simulink library "CryoDetLibCMB"  (R2016b)
settings: Solver=VariableStepAuto  StartTime=0.0  StopTime=10.0  RelTol=1e-3
values from neighbouring files (symbols this model uses):
  Fclk = Fadc    (= 307200000)    [setupCryoFPGA.m]    (also in setupCryoFPGA_CMB.m; setupCryoFPGAorig.m = 312500000)
undefined symbols (not defined in the file or in its folder): xlipgetpartsetting
libraries: xbsIndex_r4 x255, CryoDetLibCMB x19, CryoDetLib x2, simulink x1
(part 2 of 3)

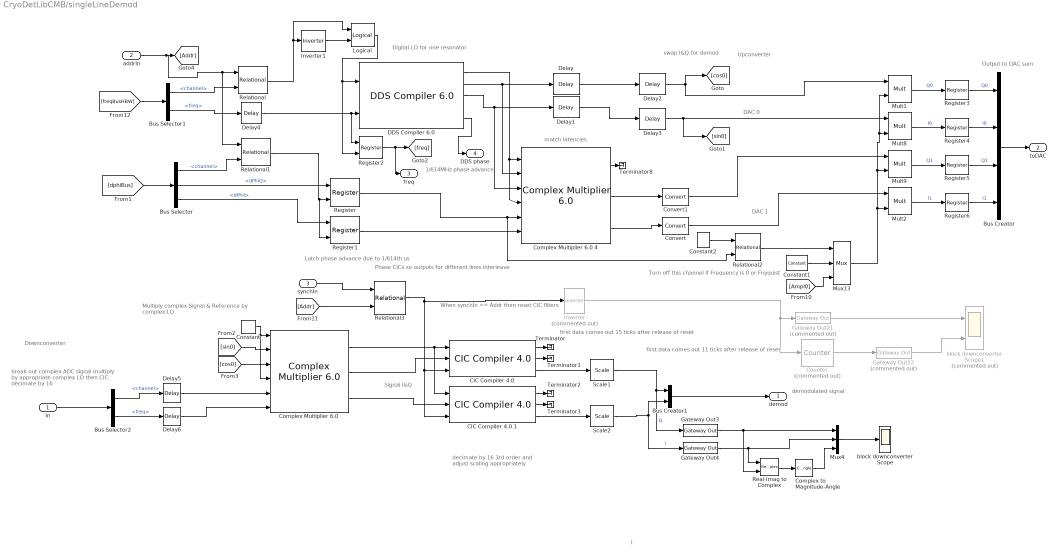
== system CryoDetLibCMB/singleLineDemod ==
  note: swap I&Q for demod
  note: Output to DAC sum
  note: decimate by 16 3rd order
      | and adjust scaling appropriately
  note: When synchIn == Addr then reset CIC filters
  note: Turn off this channel if Frequency is 0 or Fnyquist
  note: first data comes out 15 ticks after release of reset
  note: Latch phase advance due to 1/614th us
  note: I
  note: DAC 1
  note: DAC 0
  note: Downconverter
  note: demodulated signal
  note: Phase CICs so outputs for different lines interleave
  note: Signal I&Q
  note: Multiply complex Signal & Reference
      | by complex LO
  note: match latencies
  note: 1/614MHz
      | phase advance
  note: break out complex ADC signal
      | multiply by appropriate complex LO
      | then CIC decimate by 16
  note: Digital LO for one resonator
  note: Upconverter
  note: first data comes out 11 ticks after release of reset
  In : Inport
  addrIn : Inport  Port=2
  synchIn : Inport  Port=3
  Bus Creator : BusCreator  Inputs=4
  Bus Creator1 : BusCreator  Inputs=2
  Bus Selector : BusSelector  OutputSignals=channel,dPhiQ,dPhiI
  Bus Selector1 : BusSelector  OutputSignals=channel,freq
  Bus Selector2 : BusSelector  OutputSignals=channel,freq
  "CIC Compiler 4.0 " : xbsIndex_r4/CIC Compiler 4.0   filter_type=Decimation  number_of_stages=3  differential_delay=1  number_of_channels=1  sample_rate_changes=Fixed  fixed_or_initial_rate=16  minimum_rate=16  maximum_rate=16  ratespecification=Sample_Period  sampleperiod=1  hardwareoversamplingrate=1  quantization=Truncation  output_data_width=20  use_xtreme_dsp_slice=off  use_streaming_interface=on  has_aclken=off  has_aresetn=on  has_dout_tready=off  trim_axipin_name=on  gui_behaviour=Sysgen_GUI  input_data_width=18  ip_name=CIC Compiler  ip_version=4.0  dsptool_ready=true  wrapper_available=true  port_translation_map={ 'aclken' => 'en', 'aresetn' => 'rst' }  ipcore_xco_need_fpga_part=true  ipcore_verbose=false  block_type=cic_compiler_v4_0
  CIC Compiler 4.0 1 : xbsIndex_r4/CIC Compiler 4.0   filter_type=Decimation  number_of_stages=3  differential_delay=1  number_of_channels=1  sample_rate_changes=Fixed  fixed_or_initial_rate=16  minimum_rate=16  maximum_rate=16  ratespecification=Sample_Period  sampleperiod=1  hardwareoversamplingrate=1  quantization=Truncation  output_data_width=20  use_xtreme_dsp_slice=off  use_streaming_interface=on  has_aclken=off  has_aresetn=on  has_dout_tready=off  trim_axipin_name=on  gui_behaviour=Sysgen_GUI  input_data_width=18  ip_name=CIC Compiler  ip_version=4.0  dsptool_ready=true  wrapper_available=true  port_translation_map={ 'aclken' => 'en', 'aresetn' => 'rst' }  ipcore_xco_need_fpga_part=true  ipcore_verbose=false  block_type=cic_compiler_v4_0
  "Complex Multiplier 6.0 " : xbsIndex_r4/Complex Multiplier 6.0   hasatlast=off  hasatuser=off  atuserwidth=1  hasbtlast=off  hasbtuser=off  btuserwidth=1  multtype=Use_Mults  optimizegoal=Resources  flowcontrol=NonBlocking  outputwidth=18  roundmode=Truncate  hasctrltlast=off  hasctrltuser=off  ctrltuserwidth=1  outtlastbehv=Null  latencyconfig=Automatic  minimumlatency=37  aclken=off  aresetn=off  trim_axipin_name=on  simulation_type=hybrid_sim  simulation_model=sysgen:cmpy_v6_0  data_path_portlist={ 's_axis_a_tdata_real', 's_axis_a_tdata_imag', 's_axis_b_tdata_real', 's_axis_b_tdata_imag', 's_axis_ctrl_tdata_rounding_bit', 'm_axis_dout_tdata_real', 'm_axis_dout_tdata_imag' }  aportwidth=63  bportwidth=63  ip_name=Complex Multiplier  ip_version=6.0  dsptool_ready=true  ipcore_usecache=true  ipcore_useipmodelcache=true  ipcore_verbose=false  ipcore_latency_parameter='minimumlatency'  wrapper_available=true  port_translation_map={ 'aclken' => 'en', 'aresetn' => 'rst'}  block_type=cmpy_v6_0
  Complex Multiplier 6.0 4 : xbsIndex_r4/Complex Multiplier 6.0   hasatlast=off  hasatuser=off  atuserwidth=1  hasbtlast=off  hasbtuser=off  btuserwidth=1  multtype=Use_Mults  optimizegoal=Resources  flowcontrol=NonBlocking  outputwidth=19  roundmode=Truncate  hasctrltlast=off  hasctrltuser=off  ctrltuserwidth=1  outtlastbehv=Null  latencyconfig=Manual  minimumlatency=6  aclken=off  aresetn=off  trim_axipin_name=on  simulation_type=hybrid_sim  simulation_model=sysgen:cmpy_v6_0  data_path_portlist={ 's_axis_a_tdata_real', 's_axis_a_tdata_imag', 's_axis_b_tdata_real', 's_axis_b_tdata_imag', 's_axis_ctrl_tdata_rounding_bit', 'm_axis_dout_tdata_real', 'm_axis_dout_tdata_imag' }  aportwidth=63  bportwidth=63  ip_name=Complex Multiplier  ip_version=6.0  dsptool_ready=true  ipcore_usecache=true  ipcore_useipmodelcache=true  ipcore_verbose=false  ipcore_latency_parameter='minimumlatency'  wrapper_available=true  port_translation_map={ 'aclken' => 'en', 'aresetn' => 'rst'}  block_type=cmpy_v6_0
  Complex to Magnitude-Angle : ComplexToMagnitudeAngle  Output=Magnitude
  Constant : xbsIndex_r4/Constant  const=1  gui_display_data_type=Boolean  arith_type=Boolean  n_bits=16  bin_pt=14  preci_type=Single  exp_width=8  frac_width=24  explicit_period=off  period=1  equ=P=C  opselect=C  inp2=PCIN>>17  opr=+  inp1=P  carry=CIN  dbl_ovrd=off  block_type=constant
  Constant1 : xbsIndex_r4/Constant  const=0  gui_display_data_type=Fixed-point  arith_type=Unsigned  n_bits=16  bin_pt=16  preci_type=Single  exp_width=8  frac_width=24  explicit_period=off  period=1  equ=P=C  opselect=C  inp2=PCIN>>17  opr=+  inp1=P  carry=CIN  dbl_ovrd=off  block_type=constant
  Constant2 : xbsIndex_r4/Constant  const=0  gui_display_data_type=Fixed-point  arith_type=Unsigned  n_bits=16  bin_pt=16  preci_type=Single  exp_width=8  frac_width=24  explicit_period=off  period=1  equ=P=C  opselect=C  inp2=PCIN>>17  opr=+  inp1=P  carry=CIN  dbl_ovrd=off  block_type=constant
  Convert : xbsIndex_r4/Convert  gui_display_data_type=Fixed-point  arith_type="Signed  (2's comp)"  n_bits=16  bin_pt=14  float_type=Single  exp_bits=8  fraction_bits=24  quantization=Truncate  overflow=Saturate  en=off  latency=1  pipeline=off  dbl_ovrd=off  block_type=convert
  Convert1 : xbsIndex_r4/Convert  gui_display_data_type=Fixed-point  arith_type="Signed  (2's comp)"  n_bits=16  bin_pt=14  float_type=Single  exp_bits=8  fraction_bits=24  quantization=Truncate  overflow=Saturate  en=off  latency=1  pipeline=off  dbl_ovrd=off  block_type=convert
  Counter : xbsIndex_r4/Counter  Commented=on  cnt_type=Free Running  cnt_to=Inf  operation=Up  start_count=0  cnt_by_val=2^-8  arith_type=Unsigned  n_bits=8  bin_pt=8  load_pin=off  rst=on  en=off  explicit_period=off  period=1  use_behavioral_HDL=off  implementation=Fabric  dbl_ovrd=off  block_type=counter
  "DDS Compiler 6.0 " : xbsIndex_r4/DDS Compiler 6.0   partspresent=Phase_Generator_and_SIN_COS_LUT  dds_clock_rate=Fclk/1e6  channels=1  mode_of_operation=Standard  modulus=9  parameter_entry=Hardware_Parameters  spurious_free_dynamic_range=45  frequency_resolution=0.4  noise_shaping=None  phase_width=freqBits  output_width=IQbits  output_selection=Sine_and_Cosine  negative_sine=off  negative_cosine=off  amplitude_mode=Unit_Circle  memory_type=Auto  optimization_goal=Speed  dsp48_use=Maximal  resync=off  latency_configuration=Configurable  latency=15  has_phase_out=on  has_aclken=off  has_aresetn=off  explicit_period=on  period=Tclk  data_has_tlast=Not_Required  has_tready=off  s_phase_has_tuser=Not_Required  m_data_has_tuser=Not_Required  m_phase_has_tuser=Not_Required  s_phase_tuser_width=1  output_form=Twos_Complement  s_config_sync_mode=On_Vector  phase_increment=Programmable  output_frequency1=0  output_frequency2=0  output_frequency3=0  output_frequency4=0  output_frequency5=0  output_frequency6=0  output_frequency7=0  output_frequency8=0  output_frequency9=0  output_frequency10=0  output_frequency11=0  output_frequency12=0  output_frequency13=0  output_frequency14=0  output_frequency15=0  output_frequency16=0  pinc1='0'  pinc2='0'  pinc3='0'  pinc4='0'  pinc5='0'  pinc6='0'  pinc7='0'  pinc8='0'  pinc9='0'  pinc10='0'  pinc11='0'  pinc12='0'  pinc13='0'  pinc14='0'  pinc15='0'  pinc16='0'  phase_offset=None  phase_offset_angles1=0  phase_offset_angles2=0  phase_offset_angles3=0  phase_offset_angles4=0  phase_offset_angles5=0  phase_offset_angles6=0  phase_offset_angles7=0  phase_offset_angles8=0  phase_offset_angles9=0  phase_offset_angles10=0  phase_offset_angles11=0  phase_offset_angles12=0  phase_offset_angles13=0  phase_offset_angles14=0  phase_offset_angles15=0  phase_offset_angles16=0  poff1='0'  poff2='0'  poff3='0'  poff4='0'  poff5='0'  poff6='0'  poff7='0'  poff8='0'  poff9='0'  poff10='0'  poff11='0'  poff12='0'  poff13='0'  poff14='0'  poff15='0'  poff16='0'  trim_axipin_name=on  simulation_type=hybrid_sim  simulation_model=sysgen:xddsv6_0_cmodel  data_path_portlist={ 's_axis_config_tdata_poff', 's_axis_config_tdata_chan0_poff', 's_axis_config_tdata_pinc', 's_axis_config_tdata_chan0_pinc', 's_axis_phase_tdata_resync', 's_axis_phase_tdata_chan0_resync', 's_axis_phase_tdata_poff', 's_axis_phase_tdata_chan0_poff', 's_axis_phase_tdata_pinc', 's_axis_phase_tdata_chan0_pinc', 's_axis_phase_tdata_phase_in', 'm_axis_data_tdata_sine', 'm_axis_data_tdata_chan0_sine', 'm_axis_data_tdata_cosine', 'm_axis_data_tdata_chan0_cosine', 'm_axis_phase_tdata_phase_out', 'm_axis_phase_tdata_chan0_phase_out'}  por_mode=false  gui_behaviour=Sysgen  ip_name=DDS Compiler  ip_version=6.0  dsptool_ready=true  wrapper_available=true  port_translation_map={ 'aclken' => 'en', 'aresetn' => 'rst' }  ipcore_usecache=true  ipcore_useipmodelcache=true  ipcore_xco_need_fpga_part=true  ipcore_fpga_part=xlipgetpartsetting(gcb, {'kintex7', 'xc7k325t', '-3', 'fbg676'})  ipcore_verbose=false  block_type=dds_compiler_v6_0
  Delay : xbsIndex_r4/Delay  rst=off  infoeditControl=Selection of Reset will increase slice count due to use of real FFs and instead of SRLs  en=off  latency=6  reg_retiming=off  dbl_ovrd=off  block_type=delay
  Delay1 : xbsIndex_r4/Delay  rst=off  infoeditControl=Selection of Reset will increase slice count due to use of real FFs and instead of SRLs  en=off  latency=6  reg_retiming=off  dbl_ovrd=off  block_type=delay
  Delay2 : xbsIndex_r4/Delay  rst=off  infoeditControl=Selection of Reset will increase slice count due to use of real FFs and instead of SRLs  en=off  latency=1  reg_retiming=off  dbl_ovrd=off  block_type=delay
  Delay3 : xbsIndex_r4/Delay  rst=off  infoeditControl=Selection of Reset will increase slice count due to use of real FFs and instead of SRLs  en=off  latency=1  reg_retiming=off  dbl_ovrd=off  block_type=delay
  Delay4 : xbsIndex_r4/Delay  rst=off  infoeditControl=Selection of Reset will increase slice count due to use of real FFs and instead of SRLs  en=off  latency=2  reg_retiming=on  dbl_ovrd=off  block_type=delay
  Delay5 : xbsIndex_r4/Delay  rst=off  infoeditControl=Selection of Reset will increase slice count due to use of real FFs and instead of SRLs  en=off  latency=2  reg_retiming=on  dbl_ovrd=off  block_type=delay
  Delay6 : xbsIndex_r4/Delay  rst=off  infoeditControl=Selection of Reset will increase slice count due to use of real FFs and instead of SRLs  en=off  latency=2  reg_retiming=on  dbl_ovrd=off  block_type=delay
  Gateway Out21 : xbsIndex_r4/Gateway Out  Commented=on  inherit_from_input=off  hdl_port=off  rows=1  columns=1  UseAsDAC=off  DACChannel='1'  interface=None  automatic_assignment=on  address_offset=hex2dec('00')  intf_name=''  intf_description=''  timing_constraint=None  locs_specified=off  LOCs={}  io_standard={}  block_type=gatewayout
  Gateway Out22 : xbsIndex_r4/Gateway Out  Commented=on  inherit_from_input=off  hdl_port=off  rows=1  columns=1  UseAsDAC=off  DACChannel='1'  interface=None  automatic_assignment=on  address_offset=hex2dec('00')  intf_name=''  intf_description=''  timing_constraint=None  locs_specified=off  LOCs={}  io_standard={}  block_type=gatewayout
  Gateway Out3 : xbsIndex_r4/Gateway Out  inherit_from_input=off  hdl_port=off  rows=1  columns=1  UseAsDAC=off  DACChannel='1'  interface=None  automatic_assignment=on  address_offset=hex2dec('00')  intf_name=''  intf_description=''  timing_constraint=None  locs_specified=off  LOCs={}  io_standard={}  block_type=gatewayout
  Gateway Out4 : xbsIndex_r4/Gateway Out  inherit_from_input=off  hdl_port=off  rows=1  columns=1  UseAsDAC=off  DACChannel='1'  interface=None  automatic_assignment=on  address_offset=hex2dec('00')  intf_name=''  intf_description=''  timing_constraint=None  locs_specified=off  LOCs={}  io_standard={}  block_type=gatewayout
  Inverter : xbsIndex_r4/Inverter  Commented=on  en=off  latency=0  dbl_ovrd=off  block_type=inv
  Inverter1 : xbsIndex_r4/Inverter  en=off  latency=1  dbl_ovrd=off  block_type=inv
  Logical : xbsIndex_r4/Logical  logical_function=AND  inputs=2  en=off  latency=1  precision=Full  arith_type=Unsigned  n_bits=16  bin_pt=0  align_bp=on  dbl_ovrd=off  block_type=logical
  Mult{1..2,8..9} (4 alike) : xbsIndex_r4/Mult  precision=User Defined  arith_type="Signed  (2's comp)"  n_bits=16  bin_pt=15  quantization=Truncate  overflow=Wrap  en=off  latency=3  use_behavioral_HDL=off  opt=Speed  use_embedded=on  optimum_pipeline=off  pipeline=on  dbl_ovrd=off  use_rpm=on  placement_style=Triangular  block_type=mult
  Mux13 : xbsIndex_r4/Mux  inputs=2  en=off  latency=0  precision=Full  arith_type=Unsigned  n_bits=16  bin_pt=14  quantization=Truncate  overflow=Wrap  dbl_ovrd=off  block_type=mux
  Mux4 : Mux  Inputs=3
  Real-Imag to Complex : RealImagToComplex
  Register : xbsIndex_r4/Register  init=0  rst=off  en=on  dbl_ovrd=off  block_type=register
  Register1 : xbsIndex_r4/Register  init=0  rst=off  en=on  dbl_ovrd=off  block_type=register
  Register2 : xbsIndex_r4/Register  init=0  rst=off  en=on  dbl_ovrd=off  block_type=register
  Register{3..6} (4 alike) : xbsIndex_r4/Register  init=0  rst=off  en=off  dbl_ovrd=off  block_type=register
  Relational : xbsIndex_r4/Relational  mode=a=b  op_type=Bool  en=off  latency=1  dbl_ovrd=off  block_type=relational
  Relational1 : xbsIndex_r4/Relational  mode=a=b  op_type=Bool  en=off  latency=0  dbl_ovrd=off  block_type=relational
  Relational2 : xbsIndex_r4/Relational  mode=a!=b  op_type=Ufix  en=off  latency=1  dbl_ovrd=off  block_type=relational
  Relational3 : xbsIndex_r4/Relational  mode=a!=b  op_type=Bool  en=off  latency=0  dbl_ovrd=off  block_type=relational
  Scale1 : xbsIndex_r4/Scale  scale_factor=-12  dbl_ovrd=off  block_type=scale
  Scale2 : xbsIndex_r4/Scale  scale_factor=-12  dbl_ovrd=off  block_type=scale
  Terminator{,1..3,8} (5 alike) : Terminator
  block downconverter Scope : Scope
  block downconverter Scope1 : Scope  Commented=on  NumInputPorts=2
  demod : Outport
  toDAC : Outport  Port=2
  freq : Outport  Port=3
  DDS phase : Outport  Port=4
  wires:
  Relational/1 -> Logical/1, Inverter1/1
  Bus Selector1/1 -> Relational/2  "<channel>"
  Bus Selector1/2 -> Delay4/1  "<freq>"
  addrIn/1 -> Relational1/1, Relational/1, [Addr]
  "DDS Compiler 6.0 "/2 -> Complex Multiplier 6.0 4/2, Delay/1
  "DDS Compiler 6.0 "/3 -> Complex Multiplier 6.0 4/3, Delay1/1
  In/1 -> Bus Selector2/1
  Relational1/1 -> Register1/2, Register/2
  Register1/1 -> Complex Multiplier 6.0 4/6
  Register/1 -> Relational2/2, Complex Multiplier 6.0 4/5
  "DDS Compiler 6.0 "/1 -> Complex Multiplier 6.0 4/1, Complex Multiplier 6.0 4/4
  Delay/1 -> Delay2/1
  Delay1/1 -> Delay3/1
  [sin0] -> "Complex Multiplier 6.0 "/2
  [cos0] -> "Complex Multiplier 6.0 "/3
  "Complex Multiplier 6.0 "/2 -> "CIC Compiler 4.0 "/2
  "CIC Compiler 4.0 "/3 -> Scale1/1
  CIC Compiler 4.0 1/3 -> Scale2/1
  "Complex Multiplier 6.0 "/1 -> "CIC Compiler 4.0 "/1, CIC Compiler 4.0 1/1
  "CIC Compiler 4.0 "/1 -> Terminator/1
  CIC Compiler 4.0 1/1 -> Terminator2/1
  CIC Compiler 4.0 1/2 -> Terminator3/1
  Complex Multiplier 6.0 4/1 -> Terminator8/1
  Bus Creator/1 -> toDAC/1
  Bus Selector/2 -> Register/1  "<dPhiQ>"
  Bus Selector/3 -> Register1/1  "<dPhiI>"
  [dphiBus] -> Bus Selector/1
  Bus Selector/1 -> Relational1/2  "<channel>"
  Complex Multiplier 6.0 4/3 -> Convert/1
  Complex Multiplier 6.0 4/2 -> Convert1/1
  Constant1/1 -> Mux13/2
  [Ampl0] -> Mux13/3
  Mux13/1 -> Mult2/2, Mult9/2, Mult1/2, Mult8/2
  Constant2/1 -> Relational2/1
  Relational2/1 -> Mux13/1
  Relational3/1 -> Inverter/1, CIC Compiler 4.0 1/3, "CIC Compiler 4.0 "/3
  [Addr] -> Relational3/2
  synchIn/1 -> Relational3/1
  "CIC Compiler 4.0 "/2 -> Terminator1/1
  [freqBusHBW] -> Bus Selector1/1
  Convert1/1 -> Mult9/1
  Delay3/1 -> [sin0], Mult8/1
  Delay2/1 -> Mult1/1, [cos0]
  Delay4/1 -> Register2/1, "DDS Compiler 6.0 "/2
  Inverter1/1 -> Logical/2
  Logical/1 -> Register2/2, "DDS Compiler 6.0 "/1
  "Complex Multiplier 6.0 "/3 -> CIC Compiler 4.0 1/2
  Constant/1 -> "Complex Multiplier 6.0 "/4, "Complex Multiplier 6.0 "/1
  Convert/1 -> Mult2/1
  Mult2/1 -> Register6/1  "I1"
  Mult9/1 -> Register5/1  "Q1"
  Mult8/1 -> Register4/1  "I0"
  Mult1/1 -> Register3/1  "Q0"
  Bus Creator1/1 -> demod/1
  Scale1/1 -> Gateway Out3/1, Bus Creator1/1  "Q"
  Scale2/1 -> Gateway Out4/1, Bus Creator1/2  "I"
  Gateway Out4/1 -> Mux4/2, Real-Imag to Complex/1
  Gateway Out3/1 -> Mux4/1, Real-Imag to Complex/2
  Mux4/1 -> block downconverter Scope/1
  Gateway Out22/1 -> block downconverter Scope1/2
  Complex to Magnitude-Angle/1 -> Mux4/3
  Gateway Out21/1 -> block downconverter Scope1/1
  Counter/1 -> Gateway Out22/1
  Inverter/1 -> Counter/1, Gateway Out21/1
  Real-Imag to Complex/1 -> Complex to Magnitude-Angle/1
  Register2/1 -> freq/1, [freq]
  Delay6/1 -> "Complex Multiplier 6.0 "/6
  Delay5/1 -> "Complex Multiplier 6.0 "/5
  Register3/1 -> Bus Creator/1  "Q0"
  Register4/1 -> Bus Creator/2  "I0"
  Register5/1 -> Bus Creator/3  "Q1"
  Register6/1 -> Bus Creator/4  "I1"
  "DDS Compiler 6.0 "/5 -> DDS phase/1
  Bus Selector2/2 -> Delay6/1  "<freq>"
  Bus Selector2/1 -> Delay5/1  "<channel>"

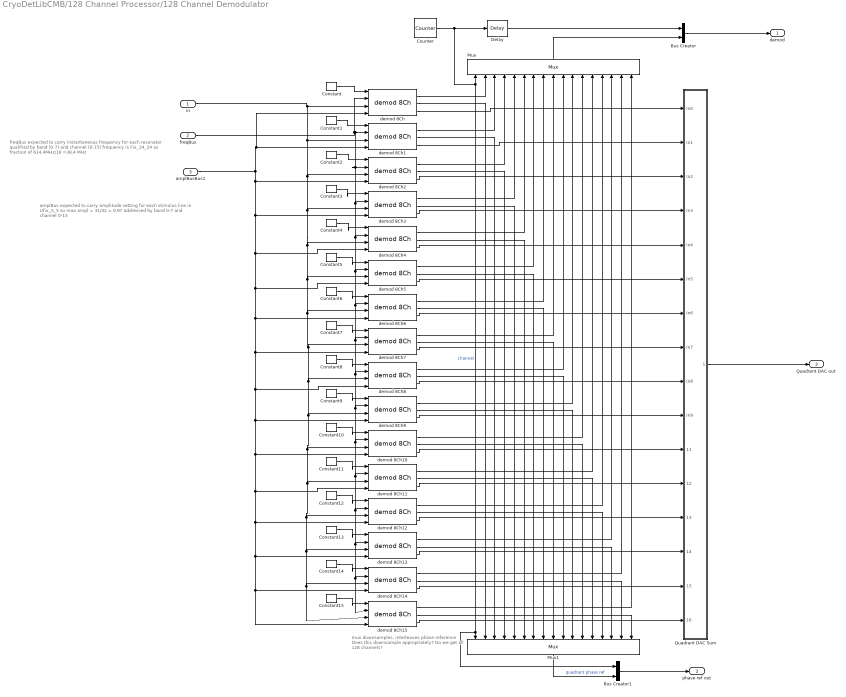
== system CryoDetLibCMB/128 Channel Processor/128 Channel Demodulator ==
  note: amplBus expected to carry  amplitude setting for each stimulus line
      | in Ufix_5_5 so max ampl = 31/32 = 0.97
      | addressed by band 0-7 and channel 0-15
  note: freqBus expected to carry instantaneous frequency for each resonator
      | qualified by band (0-7) and channel (0-15)
      | frequency is Fix_24_24 as fraction of 614.4MHz/16 =38.4 MHz
  note: mux downsamples, interleaves phase reference
      | Does this downsample appropriately?
      | Do we get all 128 channels?
  in : Inport
  freqBus : Inport  Port=2
  amplBusBus1 : Inport  Port=3
  Bus Creator : BusCreator  Inputs=2
  Bus Creator1 : BusCreator  Inputs=2
  Constant : xbsIndex_r4/Constant  const=0  gui_display_data_type=Fixed-point  arith_type=Unsigned  n_bits=4  bin_pt=0  preci_type=Single  exp_width=8  frac_width=24  explicit_period=off  period=1  equ=P=C  opselect=C  inp2=PCIN>>17  opr=+  inp1=P  carry=CIN  dbl_ovrd=off  block_type=constant
  Constant1 : xbsIndex_r4/Constant  const=1  gui_display_data_type=Fixed-point  arith_type=Unsigned  n_bits=4  bin_pt=0  preci_type=Single  exp_width=8  frac_width=24  explicit_period=off  period=1  equ=P=C  opselect=C  inp2=PCIN>>17  opr=+  inp1=P  carry=CIN  dbl_ovrd=off  block_type=constant
  Constant10 : xbsIndex_r4/Constant  const=10  gui_display_data_type=Fixed-point  arith_type=Unsigned  n_bits=4  bin_pt=0  preci_type=Single  exp_width=8  frac_width=24  explicit_period=off  period=1  equ=P=C  opselect=C  inp2=PCIN>>17  opr=+  inp1=P  carry=CIN  dbl_ovrd=off  block_type=constant
  Constant11 : xbsIndex_r4/Constant  const=11  gui_display_data_type=Fixed-point  arith_type=Unsigned  n_bits=4  bin_pt=0  preci_type=Single  exp_width=8  frac_width=24  explicit_period=off  period=1  equ=P=C  opselect=C  inp2=PCIN>>17  opr=+  inp1=P  carry=CIN  dbl_ovrd=off  block_type=constant
  Constant12 : xbsIndex_r4/Constant  const=12  gui_display_data_type=Fixed-point  arith_type=Unsigned  n_bits=4  bin_pt=0  preci_type=Single  exp_width=8  frac_width=24  explicit_period=off  period=1  equ=P=C  opselect=C  inp2=PCIN>>17  opr=+  inp1=P  carry=CIN  dbl_ovrd=off  block_type=constant
  Constant13 : xbsIndex_r4/Constant  const=13  gui_display_data_type=Fixed-point  arith_type=Unsigned  n_bits=4  bin_pt=0  preci_type=Single  exp_width=8  frac_width=24  explicit_period=off  period=1  equ=P=C  opselect=C  inp2=PCIN>>17  opr=+  inp1=P  carry=CIN  dbl_ovrd=off  block_type=constant
  Constant14 : xbsIndex_r4/Constant  const=14  gui_display_data_type=Fixed-point  arith_type=Unsigned  n_bits=4  bin_pt=0  preci_type=Single  exp_width=8  frac_width=24  explicit_period=off  period=1  equ=P=C  opselect=C  inp2=PCIN>>17  opr=+  inp1=P  carry=CIN  dbl_ovrd=off  block_type=constant
  Constant15 : xbsIndex_r4/Constant  const=15  gui_display_data_type=Fixed-point  arith_type=Unsigned  n_bits=4  bin_pt=0  preci_type=Single  exp_width=8  frac_width=24  explicit_period=off  period=1  equ=P=C  opselect=C  inp2=PCIN>>17  opr=+  inp1=P  carry=CIN  dbl_ovrd=off  block_type=constant
  Constant2 : xbsIndex_r4/Constant  const=2  gui_display_data_type=Fixed-point  arith_type=Unsigned  n_bits=4  bin_pt=0  preci_type=Single  exp_width=8  frac_width=24  explicit_period=off  period=1  equ=P=C  opselect=C  inp2=PCIN>>17  opr=+  inp1=P  carry=CIN  dbl_ovrd=off  block_type=constant
  Constant3 : xbsIndex_r4/Constant  const=3  gui_display_data_type=Fixed-point  arith_type=Unsigned  n_bits=4  bin_pt=0  preci_type=Single  exp_width=8  frac_width=24  explicit_period=off  period=1  equ=P=C  opselect=C  inp2=PCIN>>17  opr=+  inp1=P  carry=CIN  dbl_ovrd=off  block_type=constant
  Constant4 : xbsIndex_r4/Constant  const=4  gui_display_data_type=Fixed-point  arith_type=Unsigned  n_bits=4  bin_pt=0  preci_type=Single  exp_width=8  frac_width=24  explicit_period=off  period=1  equ=P=C  opselect=C  inp2=PCIN>>17  opr=+  inp1=P  carry=CIN  dbl_ovrd=off  block_type=constant
  Constant5 : xbsIndex_r4/Constant  const=5  gui_display_data_type=Fixed-point  arith_type=Unsigned  n_bits=4  bin_pt=0  preci_type=Single  exp_width=8  frac_width=24  explicit_period=off  period=1  equ=P=C  opselect=C  inp2=PCIN>>17  opr=+  inp1=P  carry=CIN  dbl_ovrd=off  block_type=constant
  Constant6 : xbsIndex_r4/Constant  const=6  gui_display_data_type=Fixed-point  arith_type=Unsigned  n_bits=4  bin_pt=0  preci_type=Single  exp_width=8  frac_width=24  explicit_period=off  period=1  equ=P=C  opselect=C  inp2=PCIN>>17  opr=+  inp1=P  carry=CIN  dbl_ovrd=off  block_type=constant
  Constant7 : xbsIndex_r4/Constant  const=7  gui_display_data_type=Fixed-point  arith_type=Unsigned  n_bits=4  bin_pt=0  preci_type=Single  exp_width=8  frac_width=24  explicit_period=off  period=1  equ=P=C  opselect=C  inp2=PCIN>>17  opr=+  inp1=P  carry=CIN  dbl_ovrd=off  block_type=constant
  Constant8 : xbsIndex_r4/Constant  const=8  gui_display_data_type=Fixed-point  arith_type=Unsigned  n_bits=4  bin_pt=0  preci_type=Single  exp_width=8  frac_width=24  explicit_period=off  period=1  equ=P=C  opselect=C  inp2=PCIN>>17  opr=+  inp1=P  carry=CIN  dbl_ovrd=off  block_type=constant
  Constant9 : xbsIndex_r4/Constant  const=9  gui_display_data_type=Fixed-point  arith_type=Unsigned  n_bits=4  bin_pt=0  preci_type=Single  exp_width=8  frac_width=24  explicit_period=off  period=1  equ=P=C  opselect=C  inp2=PCIN>>17  opr=+  inp1=P  carry=CIN  dbl_ovrd=off  block_type=constant
  Counter : xbsIndex_r4/Counter  cnt_type=Free Running  cnt_to=Inf  operation=Up  start_count=0  cnt_by_val=1  arith_type=Unsigned  n_bits=4  bin_pt=0  load_pin=off  rst=off  en=off  explicit_period=on  period=Tclk  use_behavioral_HDL=off  implementation=Fabric  dbl_ovrd=off  block_type=counter
  Delay : xbsIndex_r4/Delay  rst=off  infoeditControl=Selection of Reset will increase slice count due to use of real FFs and instead of SRLs  en=off  latency=1  reg_retiming=off  dbl_ovrd=off  block_type=delay
  Mux : xbsIndex_r4/Mux  inputs=16  en=off  latency=1  precision=Full  arith_type=Unsigned  n_bits=16  bin_pt=14  quantization=Truncate  overflow=Wrap  dbl_ovrd=off  block_type=mux
  Mux1 : xbsIndex_r4/Mux  inputs=16  en=off  latency=1  precision=Full  arith_type=Unsigned  n_bits=16  bin_pt=14  quantization=Truncate  overflow=Wrap  dbl_ovrd=off  block_type=mux
  Quadrant DAC Sum : Subsystem
  demod 8Ch{,1..15} (16 alike) : CryoDetLibCMB/demod 8Ch
  demod : Outport
  phase ref out : Outport  Port=2
  Quadrant DAC out : Outport  Port=3
  wires:
  Constant/1 -> demod 8Ch/1
  Constant1/1 -> demod 8Ch1/1
  Constant2/1 -> demod 8Ch2/1
  Constant3/1 -> demod 8Ch3/1
  Constant4/1 -> demod 8Ch4/1
  Constant5/1 -> demod 8Ch5/1
  Constant6/1 -> demod 8Ch6/1
  Constant7/1 -> demod 8Ch7/1
  Constant8/1 -> demod 8Ch8/1
  Constant9/1 -> demod 8Ch9/1
  Constant10/1 -> demod 8Ch10/1
  Constant11/1 -> demod 8Ch11/1
  Constant12/1 -> demod 8Ch12/1
  Constant13/1 -> demod 8Ch13/1
  Constant14/1 -> demod 8Ch14/1
  freqBus/1 -> demod 8Ch2/2, demod 8Ch5/2, demod 8Ch6/2, demod 8Ch7/2, demod 8Ch8/2, demod 8Ch10/2, demod 8Ch11/2, demod 8Ch12/2, demod 8Ch13/2, demod 8Ch14/2, demod 8Ch15/2, demod 8Ch9/2, demod 8Ch4/2, demod 8Ch3/2, demod 8Ch1/2, demod 8Ch/2
  demod 8Ch/1 -> Mux/2
  Counter/1 -> Delay/1, Bus Creator1/1, Mux1/1, Mux/1  "channel"
  Delay/1 -> Bus Creator/1
  Mux/1 -> Bus Creator/2
  demod 8Ch1/1 -> Mux/3
  demod 8Ch2/1 -> Mux/4
  demod 8Ch3/1 -> Mux/5
  demod 8Ch4/1 -> Mux/6
  demod 8Ch5/1 -> Mux/7
  demod 8Ch/2 -> Mux1/2
  demod 8Ch1/2 -> Mux1/3
  demod 8Ch2/2 -> Mux1/4
  demod 8Ch3/2 -> Mux1/5
  demod 8Ch4/2 -> Mux1/6
  demod 8Ch5/2 -> Mux1/7
  demod 8Ch/3 -> Quadrant DAC Sum/1(In0)
  demod 8Ch1/3 -> Quadrant DAC Sum/2(In1)
  demod 8Ch2/3 -> Quadrant DAC Sum/3(In2)
  demod 8Ch3/3 -> Quadrant DAC Sum/4(In3)
  demod 8Ch4/3 -> Quadrant DAC Sum/5(In4)
  demod 8Ch5/3 -> Quadrant DAC Sum/6(In5)
  demod 8Ch6/3 -> Quadrant DAC Sum/7(In6)
  demod 8Ch7/3 -> Quadrant DAC Sum/8(In7)
  demod 8Ch8/3 -> Quadrant DAC Sum/9(In8)
  demod 8Ch9/3 -> Quadrant DAC Sum/10(In9)
  demod 8Ch10/3 -> Quadrant DAC Sum/11(In10)
  demod 8Ch11/3 -> Quadrant DAC Sum/12(In11)
  demod 8Ch12/3 -> Quadrant DAC Sum/13(In12)
  demod 8Ch13/3 -> Quadrant DAC Sum/14(In13)
  demod 8Ch14/3 -> Quadrant DAC Sum/15(In14)
  Constant15/1 -> demod 8Ch15/1
  demod 8Ch15/3 -> Quadrant DAC Sum/16(In15)
  demod 8Ch15/2 -> Mux1/17
  demod 8Ch14/2 -> Mux1/16
  demod 8Ch13/2 -> Mux1/15
  demod 8Ch6/1 -> Mux/8
  demod 8Ch7/1 -> Mux/9
  demod 8Ch8/1 -> Mux/10
  demod 8Ch9/1 -> Mux/11
  demod 8Ch10/1 -> Mux/12
  demod 8Ch11/1 -> Mux/13
  demod 8Ch12/1 -> Mux/14
  demod 8Ch13/1 -> Mux/15
  demod 8Ch14/1 -> Mux/16
  demod 8Ch15/1 -> Mux/17
  demod 8Ch6/2 -> Mux1/8
  demod 8Ch12/2 -> Mux1/14
  demod 8Ch11/2 -> Mux1/13
  demod 8Ch10/2 -> Mux1/12
  demod 8Ch9/2 -> Mux1/11
  demod 8Ch7/2 -> Mux1/9
  demod 8Ch8/2 -> Mux1/10
  Mux1/1 -> Bus Creator1/2  "quadrant phase ref"
  Bus Creator1/1 -> phase ref out/1
  in/1 -> demod 8Ch/3, demod 8Ch2/3, demod 8Ch6/3, demod 8Ch7/3, demod 8Ch8/3, demod 8Ch10/3, demod 8Ch12/3, demod 8Ch15/3, demod 8Ch14/3, demod 8Ch13/3, demod 8Ch11/3, demod 8Ch9/3, demod 8Ch5/3, demod 8Ch4/3, demod 8Ch3/3, demod 8Ch1/3
  Bus Creator/1 -> demod/1
  Quadrant DAC Sum/1(Out2) -> Quadrant DAC out/1
  amplBusBus1/1 -> demod 8Ch/4, demod 8Ch1/4, demod 8Ch4/4, demod 8Ch5/4, demod 8Ch6/4, demod 8Ch7/4, demod 8Ch8/4, demod 8Ch9/4, demod 8Ch10/4, demod 8Ch11/4, demod 8Ch12/4, demod 8Ch13/4, demod 8Ch14/4, demod 8Ch15/4, demod 8Ch3/4, demod 8Ch2/4

== system CryoDetLibCMB/128 Channel Processor/Loop Filter ==
  In1 : Inport
  Out1 : Outport
  wires:
  In1/1 -> Out1/1

== system CryoDetLibCMB/128 Channel Processor/dF ==
  demod in : Inport
  phase ref in : Inport  Port=2
  Out1 : Outport
  wires:
  demod in/1 -> Out1/1

== system CryoDetLibCMB/demod 8Ch/CIC reset ==
  note: where N is number of channels in CIC filter
  note: reset latched resetIn
  note: latch resetIn
  note: CIC reset
      |
      | Synchronizes a CIC compiler 4.0 multi-channel CIC filter
      | to input channels
      |
      | Generates:
      | 1	notResetOut to CIC aresetn
      | 2	tlast to CIC tlast input
      |
      | Inputs:
      | 1	reset in
      | 2	Channel number (0-N) which may go to sel input of mux generating the input data stream
      | 3	N-2 which tells this module how deep is the multiplexing (e.g. N-2 = 10 for a 12 channel CIC filter (sorry))
      |
      | Guarantees:
      | 1	reset out is at least 2 clocks long
      | 2	end of reset occurs 2 clocks before channel 0
      | 3	tlast comes with channel N-1
      |
      | Assumes:
      | CIC oversampling set to "Sample period" = 1
      | No "streaming interface"
  resetIn : Inport
  Channel : Inport  Port=2
  N-2 : Inport  Port=3
  Constant : xbsIndex_r4/Constant  const=0  gui_display_data_type=Boolean  arith_type=Boolean  n_bits=16  bin_pt=14  preci_type=Single  exp_width=8  frac_width=24  explicit_period=off  period=1  equ=P=C  opselect=C  inp2=PCIN>>17  opr=+  inp1=P  carry=CIN  dbl_ovrd=off  block_type=constant
  Delay1 : xbsIndex_r4/Delay  rst=off  infoeditControl=Selection of Reset will increase slice count due to use of real FFs and instead of SRLs  en=off  latency=1  reg_retiming=off  dbl_ovrd=off  block_type=delay
  Delay2 : xbsIndex_r4/Delay  rst=off  infoeditControl=Selection of Reset will increase slice count due to use of real FFs and instead of SRLs  en=off  latency=1  reg_retiming=off  dbl_ovrd=off  block_type=delay
  Delay3 : xbsIndex_r4/Delay  rst=off  infoeditControl=Selection of Reset will increase slice count due to use of real FFs and instead of SRLs  en=off  latency=1  reg_retiming=off  dbl_ovrd=off  block_type=delay
  Inverter : xbsIndex_r4/Inverter  en=off  latency=2  dbl_ovrd=off  block_type=inv
  Inverter1 : xbsIndex_r4/Inverter  en=off  latency=0  dbl_ovrd=off  block_type=inv
  Logical : xbsIndex_r4/Logical  logical_function=AND  inputs=4  en=off  latency=0  precision=User Defined  arith_type=Boolean  n_bits=1  bin_pt=0  align_bp=on  dbl_ovrd=off  block_type=logical
  Logical1 : xbsIndex_r4/Logical  logical_function=OR  inputs=2  en=off  latency=0  precision=User Defined  arith_type=Boolean  n_bits=1  bin_pt=0  align_bp=on  dbl_ovrd=off  block_type=logical
  Mux : xbsIndex_r4/Mux  inputs=2  en=off  latency=0  precision=Full  arith_type=Unsigned  n_bits=16  bin_pt=14  quantization=Truncate  overflow=Wrap  dbl_ovrd=off  block_type=mux
  Relational1 : xbsIndex_r4/Relational  mode=a=b  op_type=Bool  en=off  latency=0  dbl_ovrd=off  block_type=relational
  notResetOut : Outport
  tlast : Outport  Port=2
  wires:
  resetIn/1 -> Inverter/1, Logical1/1
  Channel/1 -> Relational1/1
  N-2/1 -> Relational1/2
  Relational1/1 -> Logical/4, Delay1/1
  Logical1/1 -> Inverter1/1, Delay2/1
  Mux/1 -> Logical1/2
  Delay2/1 -> Logical/2, Delay3/1, Mux/2
  Constant/1 -> Mux/3
  Logical/1 -> Mux/1
  Delay1/1 -> tlast/1
  Inverter/1 -> Logical/1
  Delay3/1 -> Logical/3
  Inverter1/1 -> notResetOut/1

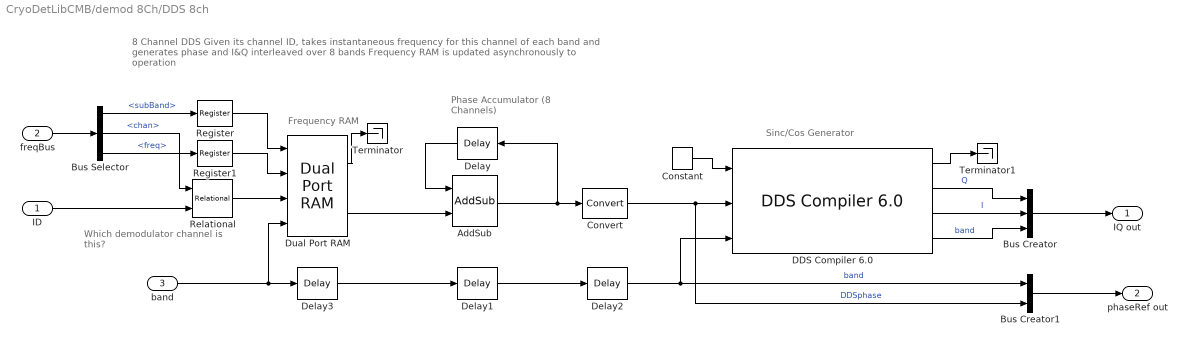
== system CryoDetLibCMB/demod 8Ch/DDS 8ch ==
  note: 8 Channel DDS
      | Given its channel ID, takes instantaneous frequency for this channel of each band and generates phase and I&Q
      | interleaved over 8 bands
      | Frequency RAM is updated asynchronously to operation
  note: Phase Accumulator
      | (8 Channels)
  note: Frequency RAM
  note: Sinc/Cos Generator
  note: Which demodulator channel is this?
  ID : Inport
  freqBus : Inport  Port=2
  band : Inport  Port=3
  AddSub : xbsIndex_r4/AddSub  mode=Addition  use_carryin=off  use_carryout=off  en=off  latency=3  precision=User Defined  arith_type=Unsigned  n_bits=24  bin_pt=24  quantization=Truncate  overflow=Wrap  use_behavioral_HDL=off  hw_selection=Fabric  pipelined=off  dbl_ovrd=off  block_type=addsub
  Bus Creator : BusCreator  Inputs=3
  Bus Creator1 : BusCreator  Inputs=2
  Bus Selector : BusSelector  OutputSignals=subBand,chan,freq
  Constant : xbsIndex_r4/Constant  const=1.0  gui_display_data_type=Boolean  arith_type=Boolean  n_bits=16  bin_pt=14  preci_type=Single  exp_width=8  frac_width=24  explicit_period=off  period=1  equ=P=C  opselect=C  inp2=PCIN>>17  opr=+  inp1=P  carry=CIN  dbl_ovrd=off  block_type=constant
  Convert : xbsIndex_r4/Convert  gui_display_data_type=Fixed-point  arith_type=Unsigned  n_bits=16  bin_pt=16  float_type=Single  exp_bits=8  fraction_bits=24  quantization=Truncate  overflow=Wrap  en=off  latency=1  pipeline=off  dbl_ovrd=off  block_type=convert
  "DDS Compiler 6.0 " : xbsIndex_r4/DDS Compiler 6.0   partspresent=SIN_COS_LUT_only  dds_clock_rate=100  channels=1  mode_of_operation=Standard  modulus=9  parameter_entry=System_Parameters  spurious_free_dynamic_range=45  frequency_resolution=0.4  noise_shaping=None  phase_width=16  output_width=16  output_selection=Sine_and_Cosine  negative_sine=off  negative_cosine=off  amplitude_mode=Unit_Circle  memory_type=Auto  optimization_goal=Auto  dsp48_use=Minimal  resync=off  latency_configuration=Auto  latency=1  has_phase_out=off  has_aclken=off  has_aresetn=off  explicit_period=off  period=1  data_has_tlast=Not_Required  has_tready=off  s_phase_has_tuser=User_Field  m_data_has_tuser=User_Field  m_phase_has_tuser=Not_Required  s_phase_tuser_width=3  output_form=Twos_Complement  s_config_sync_mode=On_Vector  phase_increment=Streaming  output_frequency1=0  output_frequency2=0  output_frequency3=0  output_frequency4=0  output_frequency5=0  output_frequency6=0  output_frequency7=0  output_frequency8=0  output_frequency9=0  output_frequency10=0  output_frequency11=0  output_frequency12=0  output_frequency13=0  output_frequency14=0  output_frequency15=0  output_frequency16=0  pinc1='0'  pinc2='0'  pinc3='0'  pinc4='0'  pinc5='0'  pinc6='0'  pinc7='0'  pinc8='0'  pinc9='0'  pinc10='0'  pinc11='0'  pinc12='0'  pinc13='0'  pinc14='0'  pinc15='0'  pinc16='0'  phase_offset=Streaming  phase_offset_angles1=0  phase_offset_angles2=0  phase_offset_angles3=0  phase_offset_angles4=0  phase_offset_angles5=0  phase_offset_angles6=0  phase_offset_angles7=0  phase_offset_angles8=0  phase_offset_angles9=0  phase_offset_angles10=0  phase_offset_angles11=0  phase_offset_angles12=0  phase_offset_angles13=0  phase_offset_angles14=0  phase_offset_angles15=0  phase_offset_angles16=0  poff1='0'  poff2='0'  poff3='0'  poff4='0'  poff5='0'  poff6='0'  poff7='0'  poff8='0'  poff9='0'  poff10='0'  poff11='0'  poff12='0'  poff13='0'  poff14='0'  poff15='0'  poff16='0'  trim_axipin_name=on  simulation_type=hybrid_sim  simulation_model=sysgen:xddsv6_0_cmodel  data_path_portlist={ 's_axis_config_tdata_poff', 's_axis_config_tdata_chan0_poff', 's_axis_config_tdata_pinc', 's_axis_config_tdata_chan0_pinc', 's_axis_phase_tdata_resync', 's_axis_phase_tdata_chan0_resync', 's_axis_phase_tdata_poff', 's_axis_phase_tdata_chan0_poff', 's_axis_phase_tdata_pinc', 's_axis_phase_tdata_chan0_pinc', 's_axis_phase_tdata_phase_in', 'm_axis_data_tdata_sine', 'm_axis_data_tdata_chan0_sine', 'm_axis_data_tdata_cosine', 'm_axis_data_tdata_chan0_cosine', 'm_axis_phase_tdata_phase_out', 'm_axis_phase_tdata_chan0_phase_out'}  por_mode=false  gui_behaviour=Sysgen  ip_name=DDS Compiler  ip_version=6.0  dsptool_ready=true  wrapper_available=true  port_translation_map={ 'aclken' => 'en', 'aresetn' => 'rst' }  ipcore_usecache=true  ipcore_useipmodelcache=true  ipcore_xco_need_fpga_part=true  ipcore_verbose=false  block_type=dds_compiler_v6_0
  Delay : xbsIndex_r4/Delay  rst=off  infoeditControl=Selection of Reset will increase slice count due to use of real FFs and instead of SRLs  en=off  latency=5  reg_retiming=off  dbl_ovrd=off  block_type=delay
  Delay1 : xbsIndex_r4/Delay  rst=off  infoeditControl=Selection of Reset will increase slice count due to use of real FFs and instead of SRLs  en=off  latency=3  reg_retiming=off  dbl_ovrd=off  block_type=delay
  Delay2 : xbsIndex_r4/Delay  rst=off  infoeditControl=Selection of Reset will increase slice count due to use of real FFs and instead of SRLs  en=off  latency=1  reg_retiming=off  dbl_ovrd=off  block_type=delay
  Delay3 : xbsIndex_r4/Delay  rst=off  infoeditControl=Selection of Reset will increase slice count due to use of real FFs and instead of SRLs  en=off  latency=1  reg_retiming=off  dbl_ovrd=off  block_type=delay
  Dual Port RAM : xbsIndex_r4/Dual Port RAM  depth=8  initVector=0  distributed_mem=Distributed memory  init_a=0  init_b=0  rst_a=off  rst_b=off  en_a=off  en_b=off  latency=1  write_mode_A=Read After Write  write_mode_B=Read After Write  optimize=Area  dbl_ovrd=off  block_type=dpram
  Register : xbsIndex_r4/Register  init=0  rst=off  en=off  dbl_ovrd=off  block_type=register
  Register1 : xbsIndex_r4/Register  init=0  rst=off  en=off  dbl_ovrd=off  block_type=register
  Relational : xbsIndex_r4/Relational  mode=a=b  op_type=Bool  en=off  latency=1  dbl_ovrd=off  block_type=relational
  Terminator : Terminator
  Terminator1 : Terminator
  IQ out : Outport
  phaseRef out : Outport  Port=2
  wires:
  Constant/1 -> "DDS Compiler 6.0 "/1
  Register1/1 -> Dual Port RAM/2
  Register/1 -> Dual Port RAM/1
  Bus Selector/2 -> Relational/1  "<chan>"
  ID/1 -> Relational/2
  Relational/1 -> Dual Port RAM/3
  Bus Selector/3 -> Register1/1  "<freq>"
  Bus Selector/1 -> Register/1  "<subBand>"
  Delay3/1 -> Delay1/1
  Delay1/1 -> Delay2/1
  Delay2/1 -> "DDS Compiler 6.0 "/3, Bus Creator1/1  "band"
  "DDS Compiler 6.0 "/1 -> Terminator1/1
  Dual Port RAM/1 -> Terminator/1
  Convert/1 -> "DDS Compiler 6.0 "/2, Bus Creator1/2  "DDSphase"
  AddSub/1 -> Convert/1, Delay/1
  band/1 -> Dual Port RAM/4, Delay3/1
  "DDS Compiler 6.0 "/2 -> Bus Creator/1  "Q"
  "DDS Compiler 6.0 "/3 -> Bus Creator/2  "I"
  "DDS Compiler 6.0 "/4 -> Bus Creator/3  "band"
  Bus Creator1/1 -> phaseRef out/1
  Bus Creator/1 -> IQ out/1
  freqBus/1 -> Bus Selector/1
  Dual Port RAM/2 -> AddSub/2
  Delay/1 -> AddSub/1

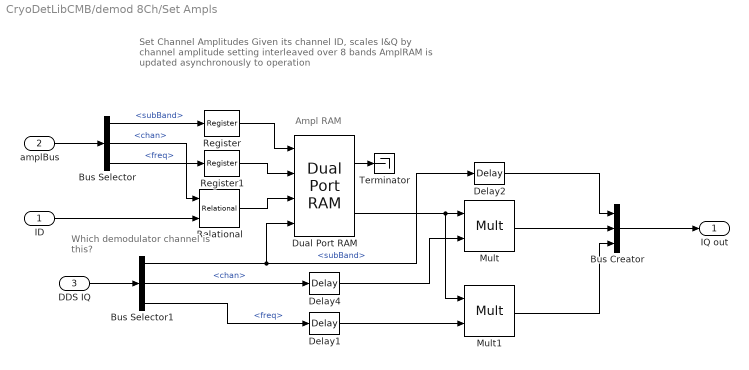
== system CryoDetLibCMB/demod 8Ch/Set Ampls ==
  note: Set Channel Amplitudes
      | Given its channel ID, scales I&Q by channel amplitude setting
      | interleaved over 8 bands
      | AmplRAM is updated asynchronously to operation
  note: Ampl RAM
  note: Which demodulator channel is this?
  ID : Inport
  amplBus : Inport  Port=2
  DDS IQ : Inport  Port=3
  Bus Creator : BusCreator  Inputs=3
  Bus Selector : BusSelector  OutputSignals=subBand,chan,freq
  Bus Selector1 : BusSelector  OutputSignals=subBand,chan,freq
  Delay1 : xbsIndex_r4/Delay  rst=off  infoeditControl=Selection of Reset will increase slice count due to use of real FFs and instead of SRLs  en=off  latency=1  reg_retiming=off  dbl_ovrd=off  block_type=delay
  Delay2 : xbsIndex_r4/Delay  rst=off  infoeditControl=Selection of Reset will increase slice count due to use of real FFs and instead of SRLs  en=off  latency=3  reg_retiming=off  dbl_ovrd=off  block_type=delay
  Delay4 : xbsIndex_r4/Delay  rst=off  infoeditControl=Selection of Reset will increase slice count due to use of real FFs and instead of SRLs  en=off  latency=1  reg_retiming=off  dbl_ovrd=off  block_type=delay
  Dual Port RAM : xbsIndex_r4/Dual Port RAM  depth=8  initVector=0  distributed_mem=Distributed memory  init_a=0  init_b=0  rst_a=off  rst_b=off  en_a=off  en_b=off  latency=1  write_mode_A=Read After Write  write_mode_B=Read After Write  optimize=Area  dbl_ovrd=off  block_type=dpram
  Mult : xbsIndex_r4/Mult  precision=User Defined  arith_type="Signed  (2's comp)"  n_bits=18  bin_pt=17  quantization=Truncate  overflow=Wrap  en=off  latency=3  use_behavioral_HDL=off  opt=Speed  use_embedded=on  optimum_pipeline=off  pipeline=on  dbl_ovrd=off  use_rpm=on  placement_style=Triangular  block_type=mult
  Mult1 : xbsIndex_r4/Mult  precision=User Defined  arith_type="Signed  (2's comp)"  n_bits=18  bin_pt=17  quantization=Truncate  overflow=Wrap  en=off  latency=3  use_behavioral_HDL=off  opt=Speed  use_embedded=on  optimum_pipeline=off  pipeline=on  dbl_ovrd=off  use_rpm=on  placement_style=Triangular  block_type=mult
  Register : xbsIndex_r4/Register  init=0  rst=off  en=off  dbl_ovrd=off  block_type=register
  Register1 : xbsIndex_r4/Register  init=0  rst=off  en=off  dbl_ovrd=off  block_type=register
  Relational : xbsIndex_r4/Relational  mode=a=b  op_type=Bool  en=off  latency=1  dbl_ovrd=off  block_type=relational
  Terminator : Terminator
  IQ out : Outport
  wires:
  Dual Port RAM/1 -> Terminator/1
  amplBus/1 -> Bus Selector/1
  Register/1 -> Dual Port RAM/1
  Bus Creator/1 -> IQ out/1
  Relational/1 -> Dual Port RAM/3
  Bus Selector/2 -> Relational/1  "<chan>"
  Bus Selector/3 -> Register1/1  "<freq>"
  Bus Selector/1 -> Register/1  "<subBand>"
  Register1/1 -> Dual Port RAM/2
  ID/1 -> Relational/2
  DDS IQ/1 -> Bus Selector1/1
  Bus Selector1/1 -> Dual Port RAM/4, Delay2/1  "<subBand>"
  Bus Selector1/2 -> Delay4/1  "<chan>"
  Bus Selector1/3 -> Delay1/1  "<freq>"
  Delay4/1 -> Mult/2
  Dual Port RAM/2 -> Mult1/1, Mult/1
  Delay1/1 -> Mult1/2
  Mult/1 -> Bus Creator/2
  Mult1/1 -> Bus Creator/3
  Delay2/1 -> Bus Creator/1

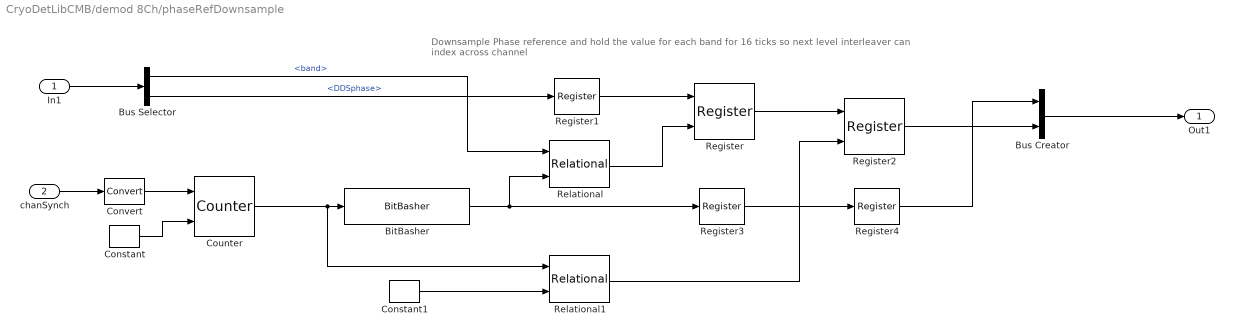
== system CryoDetLibCMB/demod 8Ch/phaseRefDownsample ==
  note: Downsample Phase reference and hold the value for each band for 16 ticks so next level interleaver can index across channel
  In1 : Inport
  chanSynch : Inport  Port=2
  BitBasher : xbsIndex_r4/BitBasher  bitexpr=band = {in[7:5]}  display_expr=on  sr_1=band  arith_type1=Unsigned  bin_pt1=0  sr_2=2  arith_type2=Unsigned  bin_pt2=0  sr_3=3  arith_type3=Unsigned  bin_pt3=0  sr_4=4  arith_type4=Unsigned  bin_pt4=0  dbl_ovrd=off  block_type=bitbasher
  Bus Creator : BusCreator  Inputs=2
  Bus Selector : BusSelector  OutputSignals=band,DDSphase
  Constant : xbsIndex_r4/Constant  const=1  gui_display_data_type=Fixed-point  arith_type=Signed (2's comp)  n_bits=7  bin_pt=0  preci_type=Single  exp_width=8  frac_width=24  explicit_period=off  period=1  equ=P=C  opselect=C  inp2=PCIN>>17  opr=+  inp1=P  carry=CIN  dbl_ovrd=off  block_type=constant
  Constant1 : xbsIndex_r4/Constant  const=0  gui_display_data_type=Fixed-point  arith_type=Signed (2's comp)  n_bits=7  bin_pt=0  preci_type=Single  exp_width=8  frac_width=24  explicit_period=off  period=1  equ=P=C  opselect=C  inp2=PCIN>>17  opr=+  inp1=P  carry=CIN  dbl_ovrd=off  block_type=constant
  Convert : xbsIndex_r4/Convert  gui_display_data_type=Boolean  arith_type=Boolean  n_bits=16  bin_pt=14  float_type=Single  exp_bits=8  fraction_bits=24  quantization=Truncate  overflow=Wrap  en=off  latency=0  pipeline=off  dbl_ovrd=off  block_type=convert
  Counter : xbsIndex_r4/Counter  cnt_type=Free Running  cnt_to=Inf  operation=Up  start_count=0  cnt_by_val=1  arith_type=Unsigned  n_bits=7  bin_pt=0  load_pin=on  rst=off  en=off  explicit_period=off  period=1  use_behavioral_HDL=off  implementation=Fabric  dbl_ovrd=off  block_type=counter
  Register : xbsIndex_r4/Register  init=0  rst=off  en=on  dbl_ovrd=off  block_type=register
  Register1 : xbsIndex_r4/Register  init=0  rst=off  en=off  dbl_ovrd=off  block_type=register
  Register2 : xbsIndex_r4/Register  init=0  rst=off  en=on  dbl_ovrd=off  block_type=register
  Register3 : xbsIndex_r4/Register  init=0  rst=off  en=off  dbl_ovrd=off  block_type=register
  Register4 : xbsIndex_r4/Register  init=0  rst=off  en=off  dbl_ovrd=off  block_type=register
  Relational : xbsIndex_r4/Relational  mode=a=b  op_type=Bool  en=off  latency=1  dbl_ovrd=off  block_type=relational
  Relational1 : xbsIndex_r4/Relational  mode=a=b  op_type=Bool  en=off  latency=1  dbl_ovrd=off  block_type=relational
  Out1 : Outport
  wires:
  In1/1 -> Bus Selector/1
  chanSynch/1 -> Convert/1
  Constant/1 -> Counter/2
  Convert/1 -> Counter/1
  Counter/1 -> Relational1/1, BitBasher/1
  BitBasher/1 -> Register3/1, Relational/2
  Bus Selector/1 -> Relational/1  "<band>"
  Relational/1 -> Register/2
  Bus Selector/2 -> Register1/1  "<DDSphase>"
  Register1/1 -> Register/1
  Constant1/1 -> Relational1/2
  Register/1 -> Register2/1
  Relational1/1 -> Register2/2
  Register2/1 -> Bus Creator/2
  Bus Creator/1 -> Out1/1
  Register3/1 -> Register4/1
  Register4/1 -> Bus Creator/1

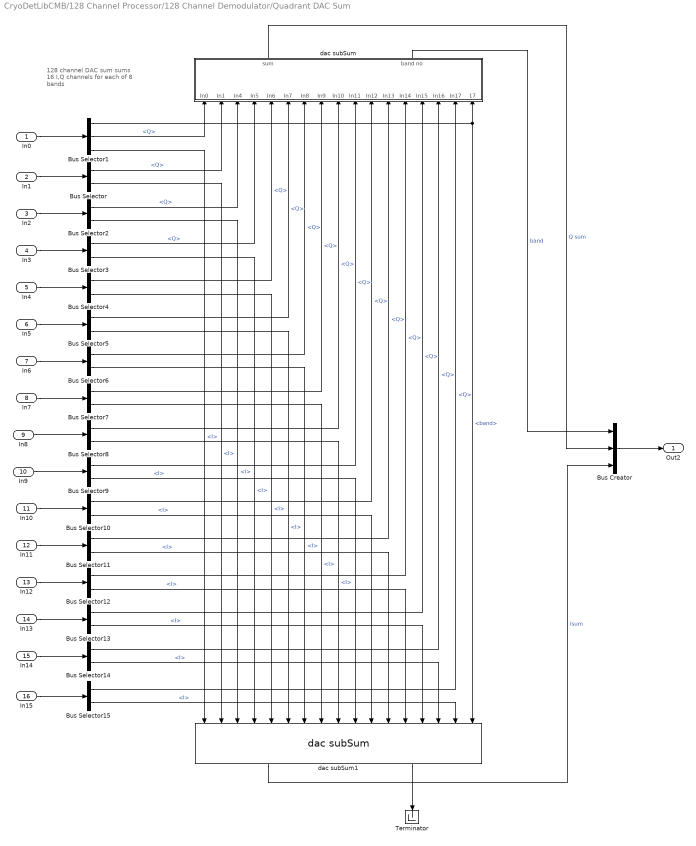
== system CryoDetLibCMB/128 Channel Processor/128 Channel Demodulator/Quadrant DAC Sum ==
  note: 128 channel DAC sum
      | sums 16 I,Q channels for each of 8 bands
  In0 : Inport
  In1 : Inport  Port=2
  In2 : Inport  Port=3
  In3 : Inport  Port=4
  In4 : Inport  Port=5
  In5 : Inport  Port=6
  In6 : Inport  Port=7
  In7 : Inport  Port=8
  In8 : Inport  Port=9
  In9 : Inport  Port=10
  In10 : Inport  Port=11
  In11 : Inport  Port=12
  In12 : Inport  Port=13
  In13 : Inport  Port=14
  In14 : Inport  Port=15
  In15 : Inport  Port=16
  Bus Creator : BusCreator  Inputs=3
  Bus Selector{,2..15} (15 alike) : BusSelector  OutputSignals=Q,I
  Bus Selector1 : BusSelector  OutputSignals=band,Q,I
  Terminator : Terminator
  dac subSum : Subsystem
  dac subSum1 : CryoDetLibCMB/128 Channel Processor/128 Channel Demodulator/Quadrant DAC Sum/dac subSum
  Out2 : Outport
  wires:
  In1/1 -> Bus Selector/1
  In0/1 -> Bus Selector1/1
  In2/1 -> Bus Selector2/1
  In3/1 -> Bus Selector3/1
  In4/1 -> Bus Selector4/1
  In5/1 -> Bus Selector5/1
  In6/1 -> Bus Selector6/1
  In7/1 -> Bus Selector7/1
  In8/1 -> Bus Selector8/1
  In9/1 -> Bus Selector9/1
  In10/1 -> Bus Selector10/1
  In11/1 -> Bus Selector11/1
  In12/1 -> Bus Selector12/1
  In13/1 -> Bus Selector13/1
  In14/1 -> Bus Selector14/1
  In15/1 -> Bus Selector15/1
  Bus Selector1/2 -> dac subSum/1(In0)  "<Q>"
  Bus Selector/1 -> dac subSum/2(In1)  "<Q>"
  Bus Selector2/1 -> dac subSum/3(In4)  "<Q>"
  Bus Selector3/1 -> dac subSum/4(In5)  "<Q>"
  Bus Selector4/1 -> dac subSum/5(In6)  "<Q>"
  Bus Selector5/1 -> dac subSum/6(In7)  "<Q>"
  Bus Selector6/1 -> dac subSum/7(In8)  "<Q>"
  Bus Selector7/1 -> dac subSum/8(In9)  "<Q>"
  Bus Selector8/1 -> dac subSum/9(In10)  "<Q>"
  Bus Selector9/1 -> dac subSum/10(In11)  "<Q>"
  Bus Selector10/1 -> dac subSum/11(In12)  "<Q>"
  Bus Selector11/1 -> dac subSum/12(In13)  "<Q>"
  Bus Selector12/1 -> dac subSum/13(In14)  "<Q>"
  Bus Selector13/1 -> dac subSum/14(In15)  "<Q>"
  Bus Selector14/1 -> dac subSum/15(In16)  "<Q>"
  Bus Selector15/1 -> dac subSum/16(In17)  "<Q>"
  Bus Selector1/1 -> dac subSum/17(band in), dac subSum1/17  "<band>"
  Bus Selector15/2 -> dac subSum1/16  "<I>"
  Bus Selector14/2 -> dac subSum1/15  "<I>"
  Bus Selector13/2 -> dac subSum1/14  "<I>"
  Bus Selector12/2 -> dac subSum1/13  "<I>"
  Bus Selector11/2 -> dac subSum1/12  "<I>"
  Bus Selector10/2 -> dac subSum1/11  "<I>"
  Bus Selector9/2 -> dac subSum1/10  "<I>"
  Bus Selector8/2 -> dac subSum1/9  "<I>"
  Bus Selector7/2 -> dac subSum1/8  "<I>"
  Bus Selector6/2 -> dac subSum1/7  "<I>"
  Bus Selector5/2 -> dac subSum1/6  "<I>"
  Bus Selector4/2 -> dac subSum1/5  "<I>"
  Bus Selector3/2 -> dac subSum1/4  "<I>"
  Bus Selector2/2 -> dac subSum1/3  "<I>"
  Bus Selector/2 -> dac subSum1/2  "<I>"
  Bus Selector1/3 -> dac subSum1/1  "<I>"
  Bus Creator/1 -> Out2/1
  dac subSum/2(band no) -> Bus Creator/1  "band"
  dac subSum/1(sum) -> Bus Creator/2  "Q sum"
  dac subSum1/1 -> Bus Creator/3  "Isum"
  dac subSum1/2 -> Terminator/1
